simulink model "gm_uz_pmsm_model_9ph_working_vnl"  (R2021a)
settings: Solver=FixedStepAuto  StartTime=0.0  StopTime=0.04  RelTol=1e-3
PreLoadFcn:
  | uz_pmsm_model_9ph_init_parameter
undefined symbols (not defined in the file or in its folder): a, b, c, friction_coefficient, inertia, k_i_d, k_p_d, k_p_q, L_d, L_o1, L_o2, L_q, L_x1, L_x2, L_y1, L_y2, L_zero, polepair, psi_pm, R_1, static_friction_torque, ts
libraries: hdlmdlgenlib x182, hdlsllib x92, simulink x15, pid_lib x2
(part 4 of 5)

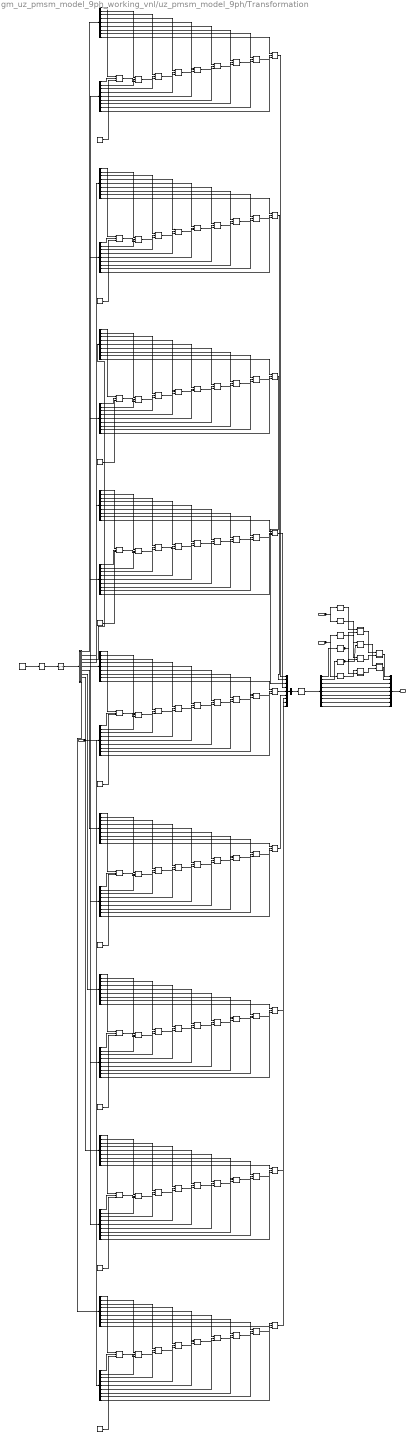
== system gm_uz_pmsm_model_9ph_working_vnl/uz_pmsm_model_9ph/Transformation ==
  in : Inport  OutDataTypeStr=fixdt(1, 25, 12)  PortDimensions=[9]  SampleTime=2e-09
  sin_theta_el : Inport  Port=2  OutDataTypeStr=single  SampleTime=2e-09
  cos_theta_el : Inport  Port=3  OutDataTypeStr=single  SampleTime=2e-09
  Add : Subsystem
      mask Display: disp('NFP\nadd');
  Add1 : Subsystem
      mask Display: disp('NFP\nadd');
  Constant1 : Constant  Value=[0.22222137451171875;0;0.22222137451171875;0;0.22222137451171875;0;0.22222137451171875;0;0.111110687255859375;-0.111110687255859375;0.1924495697021484375;0.22222137451171875;0;-0.111110687255859375;-0.1924495697021484375;-0.111110687255859375;0.1924495697021484375;0.111110687255859375;-0.111110687255859375;-0.1924495697021484375;0.22222137451171875;0;-0.111110687255859375;0.1924495697021484375;-0.111110687255859375;-0.1924495697021484375;0.111110687255859375;0.208820343017578125;0.0760040283203125;0.111110687255859375;0.1924495697021484375;-0.0385875701904296875;0.218845367431640625;-0.1702327728271484375;0.142841339111328125;-0.111110687255859375;-0.1702327728271484375;0.142841339111328125;0.111110687255859375;0.1924495697021484375;0.208820343017578125;-0.0760040283203125;-0.0385875701904296875;-0.218845367431640625;-0.111110687255859375;-0.0385875701904296875;-0.218845367431640625;0.111110687255859375;0.1924495697021484375;-0.1702327728271484375;-0.142841339111328125;0.208820343017578125;0.0760040283203125;-0.111110687255859375;0.1702327728271484375;0.142841339111328125;-0.111110687255859375;0.1924495697021484375;-0.208820343017578125;-0.0760040283203125;0.0385875701904296875;-0.218845367431640625;0.111110687255859375;-0.208820343017578125;0.0760040283203125;-0.111110687255859375;0.1924495697021484375;0.0385875701904296875;0.218845367431640625;0.1702327728271484375;0.142841339111328125;0.111110687255859375;0.0385875701904296875;-0.218845367431640625;-0.111110687255859375;0.1924495697021484375;0.1702327728271484375;-0.142841339111328125;-0.208820343017578125;0.0760040283203125;0.111110687255859375]  OutDataTypeStr=fixdt(1, 18, 19)  SampleTime=2e-09
  Data Type Conversion39 : Subsystem
      mask Display: disp('NFP\nconv');
  Data Type Conversion39_out1_0_wire : hdlmdlgenlib/Buffer
      settings: SourceProductBaseCode=SL
  Data Type Conversion39_out1_1_wire : hdlmdlgenlib/Buffer
      settings: SourceProductBaseCode=SL
  Divide : Subsystem
      mask Display: disp('NFP\nmul');
  Divide1 : Subsystem
      mask Display: disp('NFP\nmul');
  Divide2 : Subsystem
      mask Display: disp('NFP\nmul');
  Divide3 : Subsystem
      mask Display: disp('NFP\nmul');
  From{1..2,17..18} (4 alike) : hdlmdlgenlib/Buffer
      settings: SourceProductBaseCode=SL
  _adder_MultiplyAdd{,1..80} (81 alike) : hdlsllib/HDL Operations/Multiply-Add  Function=c+(a.*b)  datatype=fixdt(1, 43, 31)  DoSatur=off  FMA=off
      settings: SourceProductBaseCode=SL
  _bias{,1..8} (9 alike) : Constant  Value=double(0)  OutDataTypeStr=fixdt(1, 43, 31)  SampleTime=2e-09
  mux : Mux  Inputs=9
  t{,6..23} (19 alike) : Demux  Outputs=9
  t1 : Reshape  OutputDimensionality=Customize  OutputDimensions=[9,9]
  t2 : Math  Operator=transpose  SaturateOnIntegerOverflow=on
  t3 : Subsystem
  t4 : Mux  Inputs=9
  t5 : Concatenate  NumInputs=1  Mode=Multidimensional array  ConcatenateDimension=2
  out : Outport  SampleTime=2e-09
  wires:
  cos_theta_el/1 -> From17/1, From2/1
  sin_theta_el/1 -> From1/1, From18/1
  in/1 -> t7/1, t9/1, t11/1, t13/1, t15/1, t17/1, t19/1, t21/1, t23/1
  From1/1 -> Divide2/1(In1)
  From2/1 -> Divide3/1(In1)
  From18/1 -> Divide1/1(In1)
  From17/1 -> Divide/1(In1)
  Divide3/1(Out1) -> Add1/1(In1)
  Divide2/1(Out1) -> Add1/2(In2)
  Divide1/1(Out1) -> Add/2(In2)
  Divide/1(Out1) -> Add/1(In1)
  Data Type Conversion39/1(Out1) -> t/1
  Add1/1(Out1) -> mux/2
  Add/1(Out1) -> mux/1
  _adder_MultiplyAdd79/1 -> _adder_MultiplyAdd80/3
  t23/9 -> _adder_MultiplyAdd80/2
  t22/9 -> _adder_MultiplyAdd80/1
  _adder_MultiplyAdd78/1 -> _adder_MultiplyAdd79/3
  t23/8 -> _adder_MultiplyAdd79/2
  t22/8 -> _adder_MultiplyAdd79/1
  _adder_MultiplyAdd77/1 -> _adder_MultiplyAdd78/3
  t23/7 -> _adder_MultiplyAdd78/2
  t22/7 -> _adder_MultiplyAdd78/1
  _adder_MultiplyAdd76/1 -> _adder_MultiplyAdd77/3
  t23/6 -> _adder_MultiplyAdd77/2
  t22/6 -> _adder_MultiplyAdd77/1
  _adder_MultiplyAdd75/1 -> _adder_MultiplyAdd76/3
  t23/5 -> _adder_MultiplyAdd76/2
  t22/5 -> _adder_MultiplyAdd76/1
  _adder_MultiplyAdd74/1 -> _adder_MultiplyAdd75/3
  t23/4 -> _adder_MultiplyAdd75/2
  t22/4 -> _adder_MultiplyAdd75/1
  _adder_MultiplyAdd73/1 -> _adder_MultiplyAdd74/3
  t23/3 -> _adder_MultiplyAdd74/2
  t22/3 -> _adder_MultiplyAdd74/1
  _adder_MultiplyAdd72/1 -> _adder_MultiplyAdd73/3
  t23/2 -> _adder_MultiplyAdd73/2
  t22/2 -> _adder_MultiplyAdd73/1
  t23/1 -> _adder_MultiplyAdd72/2
  t22/1 -> _adder_MultiplyAdd72/1
  _bias8/1 -> _adder_MultiplyAdd72/3
  _adder_MultiplyAdd70/1 -> _adder_MultiplyAdd71/3
  t21/9 -> _adder_MultiplyAdd71/2
  t20/9 -> _adder_MultiplyAdd71/1
  _adder_MultiplyAdd69/1 -> _adder_MultiplyAdd70/3
  t21/8 -> _adder_MultiplyAdd70/2
  t20/8 -> _adder_MultiplyAdd70/1
  _adder_MultiplyAdd68/1 -> _adder_MultiplyAdd69/3
  t21/7 -> _adder_MultiplyAdd69/2
  t20/7 -> _adder_MultiplyAdd69/1
  _adder_MultiplyAdd67/1 -> _adder_MultiplyAdd68/3
  t21/6 -> _adder_MultiplyAdd68/2
  t20/6 -> _adder_MultiplyAdd68/1
  _adder_MultiplyAdd66/1 -> _adder_MultiplyAdd67/3
  t21/5 -> _adder_MultiplyAdd67/2
  t20/5 -> _adder_MultiplyAdd67/1
  _adder_MultiplyAdd65/1 -> _adder_MultiplyAdd66/3
  t21/4 -> _adder_MultiplyAdd66/2
  t20/4 -> _adder_MultiplyAdd66/1
  _adder_MultiplyAdd64/1 -> _adder_MultiplyAdd65/3
  t21/3 -> _adder_MultiplyAdd65/2
  t20/3 -> _adder_MultiplyAdd65/1
  _adder_MultiplyAdd63/1 -> _adder_MultiplyAdd64/3
  t21/2 -> _adder_MultiplyAdd64/2
  t20/2 -> _adder_MultiplyAdd64/1
  t21/1 -> _adder_MultiplyAdd63/2
  t20/1 -> _adder_MultiplyAdd63/1
  _bias7/1 -> _adder_MultiplyAdd63/3
  _adder_MultiplyAdd61/1 -> _adder_MultiplyAdd62/3
  t19/9 -> _adder_MultiplyAdd62/2
  t18/9 -> _adder_MultiplyAdd62/1
  _adder_MultiplyAdd60/1 -> _adder_MultiplyAdd61/3
  t19/8 -> _adder_MultiplyAdd61/2
  t18/8 -> _adder_MultiplyAdd61/1
  _adder_MultiplyAdd59/1 -> _adder_MultiplyAdd60/3
  t19/7 -> _adder_MultiplyAdd60/2
  t18/7 -> _adder_MultiplyAdd60/1
  _adder_MultiplyAdd58/1 -> _adder_MultiplyAdd59/3
  t19/6 -> _adder_MultiplyAdd59/2
  t18/6 -> _adder_MultiplyAdd59/1
  _adder_MultiplyAdd57/1 -> _adder_MultiplyAdd58/3
  t19/5 -> _adder_MultiplyAdd58/2
  t18/5 -> _adder_MultiplyAdd58/1
  _adder_MultiplyAdd56/1 -> _adder_MultiplyAdd57/3
  t19/4 -> _adder_MultiplyAdd57/2
  t18/4 -> _adder_MultiplyAdd57/1
  _adder_MultiplyAdd55/1 -> _adder_MultiplyAdd56/3
  t19/3 -> _adder_MultiplyAdd56/2
  t18/3 -> _adder_MultiplyAdd56/1
  _adder_MultiplyAdd54/1 -> _adder_MultiplyAdd55/3
  t19/2 -> _adder_MultiplyAdd55/2
  t18/2 -> _adder_MultiplyAdd55/1
  t19/1 -> _adder_MultiplyAdd54/2
  t18/1 -> _adder_MultiplyAdd54/1
  _bias6/1 -> _adder_MultiplyAdd54/3
  _adder_MultiplyAdd52/1 -> _adder_MultiplyAdd53/3
  t17/9 -> _adder_MultiplyAdd53/2
  t16/9 -> _adder_MultiplyAdd53/1
  _adder_MultiplyAdd51/1 -> _adder_MultiplyAdd52/3
  t17/8 -> _adder_MultiplyAdd52/2
  t16/8 -> _adder_MultiplyAdd52/1
  _adder_MultiplyAdd50/1 -> _adder_MultiplyAdd51/3
  t17/7 -> _adder_MultiplyAdd51/2
  t16/7 -> _adder_MultiplyAdd51/1
  _adder_MultiplyAdd49/1 -> _adder_MultiplyAdd50/3
  t17/6 -> _adder_MultiplyAdd50/2
  t16/6 -> _adder_MultiplyAdd50/1
  _adder_MultiplyAdd48/1 -> _adder_MultiplyAdd49/3
  t17/5 -> _adder_MultiplyAdd49/2
  t16/5 -> _adder_MultiplyAdd49/1
  _adder_MultiplyAdd47/1 -> _adder_MultiplyAdd48/3
  t17/4 -> _adder_MultiplyAdd48/2
  t16/4 -> _adder_MultiplyAdd48/1
  _adder_MultiplyAdd46/1 -> _adder_MultiplyAdd47/3
  t17/3 -> _adder_MultiplyAdd47/2
  t16/3 -> _adder_MultiplyAdd47/1
  _adder_MultiplyAdd45/1 -> _adder_MultiplyAdd46/3
  t17/2 -> _adder_MultiplyAdd46/2
  t16/2 -> _adder_MultiplyAdd46/1
  t17/1 -> _adder_MultiplyAdd45/2
  t16/1 -> _adder_MultiplyAdd45/1
  _bias5/1 -> _adder_MultiplyAdd45/3
  _adder_MultiplyAdd43/1 -> _adder_MultiplyAdd44/3
  t15/9 -> _adder_MultiplyAdd44/2
  t14/9 -> _adder_MultiplyAdd44/1
  _adder_MultiplyAdd42/1 -> _adder_MultiplyAdd43/3
  t15/8 -> _adder_MultiplyAdd43/2
  t14/8 -> _adder_MultiplyAdd43/1
  _adder_MultiplyAdd41/1 -> _adder_MultiplyAdd42/3
  t15/7 -> _adder_MultiplyAdd42/2
  t14/7 -> _adder_MultiplyAdd42/1
  _adder_MultiplyAdd40/1 -> _adder_MultiplyAdd41/3
  t15/6 -> _adder_MultiplyAdd41/2
  t14/6 -> _adder_MultiplyAdd41/1
  _adder_MultiplyAdd39/1 -> _adder_MultiplyAdd40/3
  t15/5 -> _adder_MultiplyAdd40/2
  t14/5 -> _adder_MultiplyAdd40/1
  _adder_MultiplyAdd38/1 -> _adder_MultiplyAdd39/3
  t15/4 -> _adder_MultiplyAdd39/2
  t14/4 -> _adder_MultiplyAdd39/1
  _adder_MultiplyAdd37/1 -> _adder_MultiplyAdd38/3
  t15/3 -> _adder_MultiplyAdd38/2
  t14/3 -> _adder_MultiplyAdd38/1
  _adder_MultiplyAdd36/1 -> _adder_MultiplyAdd37/3
  t15/2 -> _adder_MultiplyAdd37/2
  t14/2 -> _adder_MultiplyAdd37/1
  t15/1 -> _adder_MultiplyAdd36/2
  t14/1 -> _adder_MultiplyAdd36/1
  _bias4/1 -> _adder_MultiplyAdd36/3
  _adder_MultiplyAdd34/1 -> _adder_MultiplyAdd35/3
  t13/9 -> _adder_MultiplyAdd35/2
  t12/9 -> _adder_MultiplyAdd35/1
  _adder_MultiplyAdd33/1 -> _adder_MultiplyAdd34/3
  t13/8 -> _adder_MultiplyAdd34/2
  t12/8 -> _adder_MultiplyAdd34/1
  _adder_MultiplyAdd32/1 -> _adder_MultiplyAdd33/3
  t13/7 -> _adder_MultiplyAdd33/2
  t12/7 -> _adder_MultiplyAdd33/1
  _adder_MultiplyAdd31/1 -> _adder_MultiplyAdd32/3
  t13/6 -> _adder_MultiplyAdd32/2
  t12/6 -> _adder_MultiplyAdd32/1
  _adder_MultiplyAdd30/1 -> _adder_MultiplyAdd31/3
  t13/5 -> _adder_MultiplyAdd31/2
  t12/5 -> _adder_MultiplyAdd31/1
  _adder_MultiplyAdd29/1 -> _adder_MultiplyAdd30/3
  t13/4 -> _adder_MultiplyAdd30/2
  t12/4 -> _adder_MultiplyAdd30/1
  _adder_MultiplyAdd28/1 -> _adder_MultiplyAdd29/3
  t13/3 -> _adder_MultiplyAdd29/2
  t12/3 -> _adder_MultiplyAdd29/1
  _adder_MultiplyAdd27/1 -> _adder_MultiplyAdd28/3
  t13/2 -> _adder_MultiplyAdd28/2
  t12/2 -> _adder_MultiplyAdd28/1
  t13/1 -> _adder_MultiplyAdd27/2
  t12/1 -> _adder_MultiplyAdd27/1
  _bias3/1 -> _adder_MultiplyAdd27/3
  _adder_MultiplyAdd25/1 -> _adder_MultiplyAdd26/3
  t11/9 -> _adder_MultiplyAdd26/2
  t10/9 -> _adder_MultiplyAdd26/1
  _adder_MultiplyAdd24/1 -> _adder_MultiplyAdd25/3
  t11/8 -> _adder_MultiplyAdd25/2
  t10/8 -> _adder_MultiplyAdd25/1
  _adder_MultiplyAdd23/1 -> _adder_MultiplyAdd24/3
  t11/7 -> _adder_MultiplyAdd24/2
  t10/7 -> _adder_MultiplyAdd24/1
  _adder_MultiplyAdd22/1 -> _adder_MultiplyAdd23/3
  t11/6 -> _adder_MultiplyAdd23/2
  t10/6 -> _adder_MultiplyAdd23/1
  _adder_MultiplyAdd21/1 -> _adder_MultiplyAdd22/3
  t11/5 -> _adder_MultiplyAdd22/2
  t10/5 -> _adder_MultiplyAdd22/1
  _adder_MultiplyAdd20/1 -> _adder_MultiplyAdd21/3
  t11/4 -> _adder_MultiplyAdd21/2
  t10/4 -> _adder_MultiplyAdd21/1
  _adder_MultiplyAdd19/1 -> _adder_MultiplyAdd20/3
  t11/3 -> _adder_MultiplyAdd20/2
  t10/3 -> _adder_MultiplyAdd20/1
  _adder_MultiplyAdd18/1 -> _adder_MultiplyAdd19/3
  t11/2 -> _adder_MultiplyAdd19/2
  t10/2 -> _adder_MultiplyAdd19/1
  t11/1 -> _adder_MultiplyAdd18/2
  t10/1 -> _adder_MultiplyAdd18/1
  _bias2/1 -> _adder_MultiplyAdd18/3
  _adder_MultiplyAdd16/1 -> _adder_MultiplyAdd17/3
  t9/9 -> _adder_MultiplyAdd17/2
  t8/9 -> _adder_MultiplyAdd17/1
  _adder_MultiplyAdd15/1 -> _adder_MultiplyAdd16/3
  t9/8 -> _adder_MultiplyAdd16/2
  t8/8 -> _adder_MultiplyAdd16/1
  _adder_MultiplyAdd14/1 -> _adder_MultiplyAdd15/3
  t9/7 -> _adder_MultiplyAdd15/2
  t8/7 -> _adder_MultiplyAdd15/1
  _adder_MultiplyAdd13/1 -> _adder_MultiplyAdd14/3
  t9/6 -> _adder_MultiplyAdd14/2
  t8/6 -> _adder_MultiplyAdd14/1
  _adder_MultiplyAdd12/1 -> _adder_MultiplyAdd13/3
  t9/5 -> _adder_MultiplyAdd13/2
  t8/5 -> _adder_MultiplyAdd13/1
  _adder_MultiplyAdd11/1 -> _adder_MultiplyAdd12/3
  t9/4 -> _adder_MultiplyAdd12/2
  t8/4 -> _adder_MultiplyAdd12/1
  _adder_MultiplyAdd10/1 -> _adder_MultiplyAdd11/3
  t9/3 -> _adder_MultiplyAdd11/2
  t8/3 -> _adder_MultiplyAdd11/1
  _adder_MultiplyAdd9/1 -> _adder_MultiplyAdd10/3
  t9/2 -> _adder_MultiplyAdd10/2
  t8/2 -> _adder_MultiplyAdd10/1
  t9/1 -> _adder_MultiplyAdd9/2
  t8/1 -> _adder_MultiplyAdd9/1
  _bias1/1 -> _adder_MultiplyAdd9/3
  _adder_MultiplyAdd7/1 -> _adder_MultiplyAdd8/3
  t7/9 -> _adder_MultiplyAdd8/2
  t6/9 -> _adder_MultiplyAdd8/1
  _adder_MultiplyAdd6/1 -> _adder_MultiplyAdd7/3
  t7/8 -> _adder_MultiplyAdd7/2
  t6/8 -> _adder_MultiplyAdd7/1
  _adder_MultiplyAdd5/1 -> _adder_MultiplyAdd6/3
  t7/7 -> _adder_MultiplyAdd6/2
  t6/7 -> _adder_MultiplyAdd6/1
  _adder_MultiplyAdd4/1 -> _adder_MultiplyAdd5/3
  t7/6 -> _adder_MultiplyAdd5/2
  t6/6 -> _adder_MultiplyAdd5/1
  _adder_MultiplyAdd3/1 -> _adder_MultiplyAdd4/3
  t7/5 -> _adder_MultiplyAdd4/2
  t6/5 -> _adder_MultiplyAdd4/1
  _adder_MultiplyAdd2/1 -> _adder_MultiplyAdd3/3
  t7/4 -> _adder_MultiplyAdd3/2
  t6/4 -> _adder_MultiplyAdd3/1
  _adder_MultiplyAdd1/1 -> _adder_MultiplyAdd2/3
  t7/3 -> _adder_MultiplyAdd2/2
  t6/3 -> _adder_MultiplyAdd2/1
  _adder_MultiplyAdd/1 -> _adder_MultiplyAdd1/3
  t7/2 -> _adder_MultiplyAdd1/2
  t6/2 -> _adder_MultiplyAdd1/1
  t7/1 -> _adder_MultiplyAdd/2
  t6/1 -> _adder_MultiplyAdd/1
  _bias/1 -> _adder_MultiplyAdd/3
  t4/1 -> t5/1
  _adder_MultiplyAdd80/1 -> t4/9
  _adder_MultiplyAdd71/1 -> t4/8
  _adder_MultiplyAdd62/1 -> t4/7
  _adder_MultiplyAdd53/1 -> t4/6
  _adder_MultiplyAdd44/1 -> t4/5
  _adder_MultiplyAdd35/1 -> t4/4
  _adder_MultiplyAdd26/1 -> t4/3
  _adder_MultiplyAdd17/1 -> t4/2
  _adder_MultiplyAdd8/1 -> t4/1
  t3/9(out8) -> t22/1
  t3/8(out7) -> t20/1
  t3/7(out6) -> t18/1
  t3/6(out5) -> t16/1
  t3/5(out4) -> t14/1
  t3/4(out3) -> t12/1
  t3/3(out2) -> t10/1
  t3/2(out1) -> t8/1
  t3/1(out0) -> t6/1
  t2/1 -> t3/1(in0)
  Constant1/1 -> t1/1
  t/9 -> mux/9
  t/8 -> mux/8
  t/7 -> mux/7
  t/6 -> mux/6
  t/5 -> mux/5
  t/4 -> mux/4
  t/3 -> mux/3
  t/2 -> Data Type Conversion39_out1_1_wire/1
  t/1 -> Data Type Conversion39_out1_0_wire/1
  mux/1 -> out/1
  t5/1 -> Data Type Conversion39/1(In1)
  Data Type Conversion39_out1_1_wire/1 -> Divide1/2(In2), Divide3/2(In2)
  Data Type Conversion39_out1_0_wire/1 -> Divide/2(In2), Divide2/2(In2)
  t1/1 -> t2/1

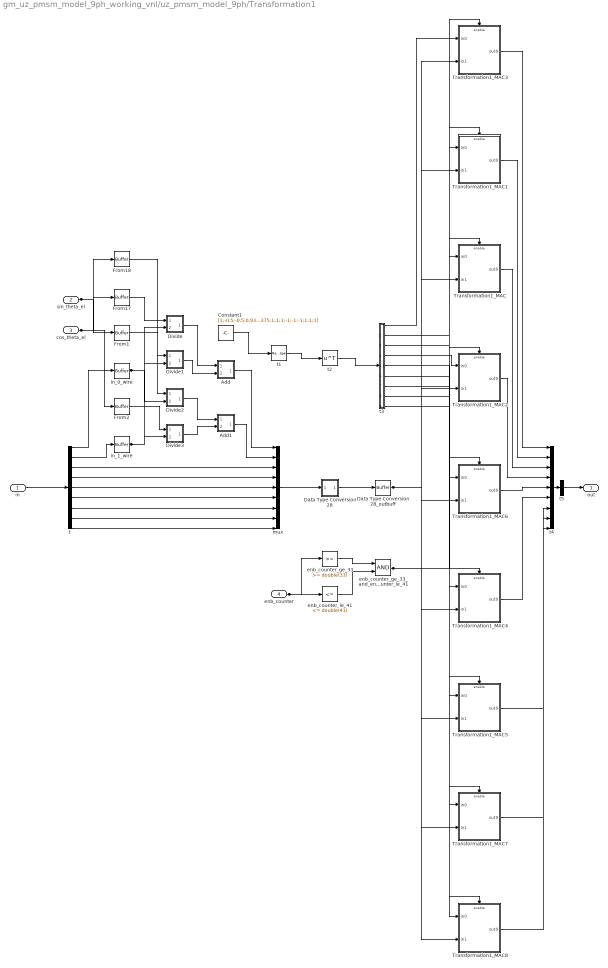
== system gm_uz_pmsm_model_9ph_working_vnl/uz_pmsm_model_9ph/Transformation1 ==
  in : Inport  OutDataTypeStr=single  PortDimensions=[9]  SampleTime=2e-09
  sin_theta_el : Inport  Port=2  OutDataTypeStr=single  SampleTime=2e-09
  cos_theta_el : Inport  Port=3  OutDataTypeStr=single  SampleTime=2e-09
  enb_counter : Inport  Port=4  OutDataTypeStr=uint16  SampleTime=2e-09
  Add : Subsystem
      mask Display: disp('NFP\nadd');
  Add1 : Subsystem
      mask Display: disp('NFP\nadd');
  Constant1 : Constant  Value=[1;-0.5;-0.5;0.939697265625;-0.7660369873046875;-0.17364501953125;0.7660369873046875;-0.939697265625;0.17364501953125;0;0.86602783203125;-0.86602783203125;0.3420257568359375;0.642791748046875;-0.98480224609375;0.642791748046875;0.3420257568359375;-0.98480224609375;1;1;1;0.5;0.5;0.5;-0.5;-0.5;-0.5;0;0;0;0.86602783203125;0.86602783203125;0.86602783203125;0.86602783203125;0.86602783203125;0.86602783203125;1;-0.5;-0.5;-0.17364501953125;0.939697265625;-0.7660369873046875;-0.939697265625;0.17364501953125;0.7660369873046875;0;-0.86602783203125;0.86602783203125;0.98480224609375;-0.3420257568359375;-0.642791748046875;-0.3420257568359375;0.98480224609375;-0.642791748046875;1;-0.5;-0.5;-0.7660369873046875;-0.17364501953125;0.939697265625;0.17364501953125;0.7660369873046875;-0.939697265625;0;0.86602783203125;-0.86602783203125;0.642791748046875;-0.98480224609375;0.3420257568359375;-0.98480224609375;0.642791748046875;0.3420257568359375;1;1;1;-1;-1;-1;1;1;1]  OutDataTypeStr=fixdt(1, 18, 16)  SampleTime=2e-09
  Data Type Conversion28 : Subsystem
      mask Display: disp('NFP\nconv');
  Data Type Conversion28_outbuff : hdlmdlgenlib/Buffer
      settings: SourceProductBaseCode=SL
  Divide : Subsystem
      mask Display: disp('NFP\nmul');
  Divide1 : Subsystem
      mask Display: disp('NFP\nmul');
  Divide2 : Subsystem
      mask Display: disp('NFP\nmul');
  Divide3 : Subsystem
      mask Display: disp('NFP\nmul');
  From{1..2,17..18} (4 alike) : hdlmdlgenlib/Buffer
      settings: SourceProductBaseCode=SL
  Transformation1_MAC : Subsystem
      settings: MinAlgLoopOccurrences=on
  Transformation1_MAC1 : Subsystem
      settings: MinAlgLoopOccurrences=on
  Transformation1_MAC2 : Subsystem
      settings: MinAlgLoopOccurrences=on
  Transformation1_MAC3 : Subsystem
      settings: MinAlgLoopOccurrences=on
  Transformation1_MAC4 : Subsystem
      settings: MinAlgLoopOccurrences=on
  Transformation1_MAC5 : Subsystem
      settings: MinAlgLoopOccurrences=on
  Transformation1_MAC6 : Subsystem
      settings: MinAlgLoopOccurrences=on
  Transformation1_MAC7 : Subsystem
      settings: MinAlgLoopOccurrences=on
  Transformation1_MAC8 : Subsystem
      settings: MinAlgLoopOccurrences=on
  enb_counter_ge_33 : simulink/Logic and Bit Operations/Compare To Constant  relop=>=  const=double(33)  OutDataTypeStr=boolean
  enb_counter_ge_33_and_enb_counter_le_41 : Logic  AllPortsSameDT=off  OutDataTypeStr=boolean  SampleTime=2e-09
  enb_counter_le_41 : simulink/Logic and Bit Operations/Compare To Constant  relop=<=  const=double(41)  OutDataTypeStr=boolean
  in_0_wire : hdlmdlgenlib/Buffer
      settings: SourceProductBaseCode=SL
  in_1_wire : hdlmdlgenlib/Buffer
      settings: SourceProductBaseCode=SL
  mux : Mux  Inputs=9
  t : Demux  Outputs=9
  t1 : Reshape  OutputDimensionality=Customize  OutputDimensions=[9,9]
  t2 : Math  Operator=transpose  SaturateOnIntegerOverflow=on
  t3 : Subsystem
  t4 : Mux  Inputs=9
  t5 : Concatenate  NumInputs=1  Mode=Multidimensional array  ConcatenateDimension=2
  out : Outport  SampleTime=2e-09
  wires:
  enb_counter/1 -> enb_counter_ge_33/1, enb_counter_le_41/1
  cos_theta_el/1 -> From17/1, From2/1
  sin_theta_el/1 -> From1/1, From18/1
  in/1 -> t/1
  enb_counter_le_41/1 -> enb_counter_ge_33_and_enb_counter_le_41/2
  enb_counter_ge_33/1 -> enb_counter_ge_33_and_enb_counter_le_41/1
  enb_counter_ge_33_and_enb_counter_le_41/1 -> Transformation1_MAC8/Enable, Transformation1_MAC7/Enable, Transformation1_MAC5/Enable, Transformation1_MAC4/Enable, Transformation1_MAC6/Enable, Transformation1_MAC2/Enable, Transformation1_MAC/Enable, Transformation1_MAC1/Enable, Transformation1_MAC3/Enable
  t3/9(out8) -> Transformation1_MAC8/1(in0)
  t3/8(out7) -> Transformation1_MAC7/1(in0)
  t3/7(out6) -> Transformation1_MAC5/1(in0)
  t3/6(out5) -> Transformation1_MAC4/1(in0)
  t3/5(out4) -> Transformation1_MAC6/1(in0)
  t3/4(out3) -> Transformation1_MAC2/1(in0)
  t3/3(out2) -> Transformation1_MAC/1(in0)
  t3/2(out1) -> Transformation1_MAC1/1(in0)
  t3/1(out0) -> Transformation1_MAC3/1(in0)
  Divide3/1(Out1) -> Add1/2(In2)
  Divide2/1(Out1) -> Add1/1(In1)
  Divide1/1(Out1) -> Add/2(In2)
  Divide/1(Out1) -> Add/1(In1)
  Data Type Conversion28/1(Out1) -> Data Type Conversion28_outbuff/1
  Add1/1(Out1) -> mux/2
  Add/1(Out1) -> mux/1
  t4/1 -> t5/1
  Transformation1_MAC8/1(out0) -> t4/9
  Transformation1_MAC7/1(out0) -> t4/8
  Transformation1_MAC5/1(out0) -> t4/7
  Transformation1_MAC4/1(out0) -> t4/6
  Transformation1_MAC6/1(out0) -> t4/5
  Transformation1_MAC2/1(out0) -> t4/4
  Transformation1_MAC/1(out0) -> t4/3
  Transformation1_MAC1/1(out0) -> t4/2
  Transformation1_MAC3/1(out0) -> t4/1
  t2/1 -> t3/1(in0)
  Constant1/1 -> t1/1
  t/9 -> mux/9
  t/8 -> mux/8
  t/7 -> mux/7
  t/6 -> mux/6
  t/5 -> mux/5
  t/4 -> mux/4
  t/3 -> mux/3
  t/2 -> in_1_wire/1
  t/1 -> in_0_wire/1
  mux/1 -> Data Type Conversion28/1(In1)
  t5/1 -> out/1
  From2/1 -> Divide3/1(In1)
  From18/1 -> Divide1/1(In1)
  From17/1 -> Divide/1(In1)
  From1/1 -> Divide2/1(In1)
  in_1_wire/1 -> Divide1/2(In2), Divide3/2(In2)
  in_0_wire/1 -> Divide/2(In2), Divide2/2(In2)
  Data Type Conversion28_outbuff/1 -> Transformation1_MAC8/2(in1), Transformation1_MAC7/2(in1), Transformation1_MAC5/2(in1), Transformation1_MAC4/2(in1), Transformation1_MAC6/2(in1), Transformation1_MAC2/2(in1), Transformation1_MAC/2(in1), Transformation1_MAC1/2(in1), Transformation1_MAC3/2(in1)
  t1/1 -> t2/1

== system gm_uz_pmsm_model_9ph_working_vnl/uz_pmsm_model_9ph_vnl/Theta_el ==
  w_mech : Inport
  polepairs : Inport  Port=2
  reset : Inport  Port=3
  Data Type Conversion1 : DataTypeConversion  OutDataTypeStr=single  RndMeth=Nearest
  Data Type Conversion2 : DataTypeConversion  OutDataTypeStr=double  RndMeth=Nearest
  Divide : Product  Inputs=**
  Mod : Math  Operator=rem  SaturateOnIntegerOverflow=on
  Pi : Constant  Value=2*pi  OutDataTypeStr=single  SampleTime=-1
  integrator8 : Subsystem
  theta_el : Outport
  wires:
  Data Type Conversion2/1 -> integrator8/1(in)
  Mod/1 -> theta_el/1  "theta_el"
  Data Type Conversion1/1 -> Mod/1
  Pi/1 -> Mod/2
  reset/1 -> integrator8/2(reset)
  integrator8/1(outt) -> Data Type Conversion1/1
  polepairs/1 -> Divide/2
  w_mech/1 -> Divide/1
  Divide/1 -> Data Type Conversion2/1

== system gm_uz_pmsm_model_9ph_working_vnl/uz_pmsm_model_9ph_vnl/Transformation ==
  in : Inport
  Add : Sum
  Add1 : Sum  Inputs=-+
  Constant1 : Constant  Value=c  OutDataTypeStr=fixdt(1,18)  SampleTime=-1
  Data Type Conversion1 : DataTypeConversion  OutDataTypeStr=single  RndMeth=Nearest
  Data Type Conversion38 : DataTypeConversion  OutDataTypeStr=single  RndMeth=Nearest
  Data Type Conversion39 : DataTypeConversion  OutDataTypeStr=single  RndMeth=Nearest
  Demux1 : Demux  Outputs=9
  Divide{,1..3} (4 alike) : Product  Inputs=**
  MatrixMultiply : Product  Multiplication=Matrix(*)
  Mux : Mux  Inputs=9
  out : Outport
  wires:
  in/1 -> MatrixMultiply/2
  Data Type Conversion39/1 -> Demux1/1
  Constant1/1 -> MatrixMultiply/1
  MatrixMultiply/1 -> Data Type Conversion39/1
  Divide2/1 -> Add1/1
  Divide3/1 -> Add1/2
  [cos_theta_el] -> Divide3/1
  [sin_theta_el] -> Divide2/1
  [cos_theta_el] -> Divide/1
  [sin_theta_el] -> Divide1/1
  Divide1/1 -> Add/2
  Divide/1 -> Add/1
  Data Type Conversion1/1 -> Divide3/2, Divide1/2  "u_beta"
  Data Type Conversion38/1 -> Divide2/2, Divide/2  "u_alpha"
  Add/1 -> Mux/1
  Add1/1 -> Mux/2
  Demux1/2 -> Data Type Conversion1/1
  Demux1/1 -> Data Type Conversion38/1
  Mux/1 -> out/1
  Demux1/9 -> Mux/9
  Demux1/8 -> Mux/8
  Demux1/7 -> Mux/7
  Demux1/6 -> Mux/6
  Demux1/5 -> Mux/5
  Demux1/4 -> Mux/4
  Demux1/3 -> Mux/3

== system gm_uz_pmsm_model_9ph_working_vnl/uz_pmsm_model_9ph_vnl/Transformation1 ==
  in : Inport
  Add : Sum  Inputs=+-
  Add1 : Sum
  Constant1 : Constant  Value=inv(c)  OutDataTypeStr=fixdt(1,18)  SampleTime=-1
  Data Type Conversion28 : DataTypeConversion  OutDataTypeStr=fixdt(1,25,12)  RndMeth=Nearest
  Demux1 : Demux  Outputs=9
  Divide{,1..3} (4 alike) : Product  Inputs=**
  MatrixMultiply : Product  Multiplication=Matrix(*)
  Mux : Mux  Inputs=9
  out : Outport
  wires:
  MatrixMultiply/1 -> out/1
  Constant1/1 -> MatrixMultiply/1
  Data Type Conversion28/1 -> MatrixMultiply/2
  Add1/1 -> Mux/2
  [cos_theta_el] -> Divide3/1
  Divide2/1 -> Add1/1
  [sin_theta_el] -> Divide2/1
  Divide3/1 -> Add1/2
  Demux1/1 -> Divide/2, Divide2/2  "i_d"
  Divide1/1 -> Add/2
  [cos_theta_el] -> Divide/1
  Divide/1 -> Add/1
  Add/1 -> Mux/1
  Demux1/2 -> Divide1/2, Divide3/2  "i_q"
  [sin_theta_el] -> Divide1/1
  Demux1/7 -> Mux/7
  Demux1/9 -> Mux/9
  Demux1/5 -> Mux/5
  Demux1/3 -> Mux/3
  Demux1/4 -> Mux/4
  Demux1/6 -> Mux/6
  Demux1/8 -> Mux/8
  Mux/1 -> Data Type Conversion28/1
  in/1 -> Demux1/1

== system gm_uz_pmsm_model_9ph_working_vnl/uz_pmsm_model_9ph_vnl/mechanical_system ==
  note: This delay breaks the algebraic loop between mechanical and electrical system.
      | Introduces a delay of 500ns.
  reset : Inport
  M_Mi : Inport  Port=2
  reciprocal_J : Inport  Port=3
  load_torque : Inport  Port=4
  Data Type Conversion1 : DataTypeConversion  OutDataTypeStr=double  RndMeth=Nearest
  Data Type Conversion8 : DataTypeConversion  OutDataTypeStr=single  RndMeth=Nearest
  Delay : Delay  DelayLength=1
  Product11 : Product
  Sum1 : Sum  Inputs=|+-
  integrator1 : Subsystem
  omega_mech : Outport
  wires:
  Data Type Conversion1/1 -> integrator1/2(in)
  Data Type Conversion8/1 -> omega_mech/1
  Delay/1 -> Sum1/1
  M_Mi/1 -> Delay/1
  load_torque/1 -> Sum1/2
  Sum1/1 -> Product11/2
  reciprocal_J/1 -> Product11/1
  reset/1 -> integrator1/1(reset)
  integrator1/1(outt) -> Data Type Conversion8/1
  Product11/1 -> Data Type Conversion1/1

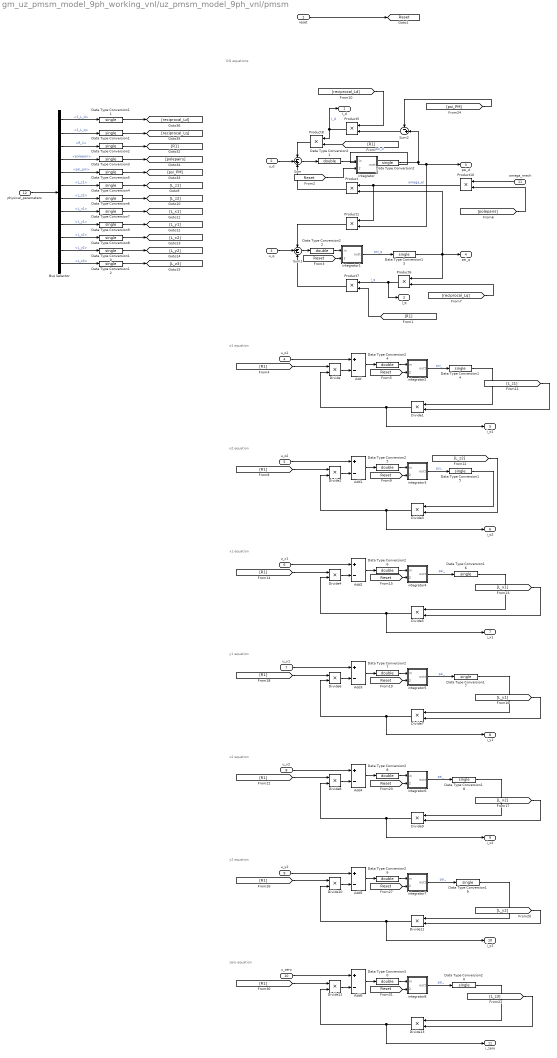
== system gm_uz_pmsm_model_9ph_working_vnl/uz_pmsm_model_9ph_vnl/pmsm ==
  note: zero equation
  note: y2 equation
  note: x2 equation
  note: y1 equation
  note: x1 equation
  note: o2 equation
  note: DQ equations
  note: o1 equation
  reset : Inport
  u_d : Inport  Port=2
  u_q : Inport  Port=3
  u_o1 : Inport  Port=4
  u_o2 : Inport  Port=5
  u_x1 : Inport  Port=6
  u_y1 : Inport  Port=7
  u_x2 : Inport  Port=8
  u_y2 : Inport  Port=9
  u_zero : Inport  Port=10
  omega_mech : Inport  Port=11
  physical_parameters : Inport  Port=12
  Add{,1..6} (7 alike) : Sum  Inputs=+-
  Bus Selector : BusSelector  OutputSignals=1_L_d,1_L_q,R_1,polepair,psi_pm,L_z1,L_z2,L_x1,L_y1,L_x2,L_y2,L_z3
  Data Type Conversion{1..20,23} (21 alike) : DataTypeConversion  OutDataTypeStr=single  RndMeth=Nearest
  Data Type Conversion{21..22,24..30} (9 alike) : DataTypeConversion  OutDataTypeStr=double  RndMeth=Nearest
  Divide{,1..13} (14 alike) : Product  Inputs=**
  Product{,1,5..8,10} (7 alike) : Product
  Sum : Sum  Inputs=-++
  Sum1 : Sum  Inputs=-+-
  Sum2 : Sum  Inputs=-+|
  integrator : Subsystem
  integrator1 : Subsystem
  integrator2 : Subsystem
  integrator3 : Subsystem
  integrator4 : Subsystem
  integrator5 : Subsystem
  integrator6 : Subsystem
  integrator7 : Subsystem
  integrator8 : Subsystem
  I_d : Outport
  I_q : Outport  Port=2
  psi_d : Outport  Port=3
  psi_q : Outport  Port=4
  i_o1 : Outport  Port=5
  i_o2 : Outport  Port=6
  i_x1 : Outport  Port=7
  i_y1 : Outport  Port=8
  i_x2 : Outport  Port=9
  i_y2 : Outport  Port=10
  i_zero : Outport  Port=11
  tag scope: Reset=global
  wires:
  Data Type Conversion30/1 -> integrator8/1(in)
  Data Type Conversion29/1 -> integrator7/1(in)
  Data Type Conversion28/1 -> integrator6/1(in)
  Data Type Conversion27/1 -> integrator5/1(in)
  Data Type Conversion26/1 -> integrator4/1(in)
  Data Type Conversion25/1 -> integrator3/1(in)
  Data Type Conversion24/1 -> integrator2/1(in)
  Data Type Conversion22/1 -> integrator1/1(in)
  Data Type Conversion21/1 -> integrator/1(in)
  Data Type Conversion20/1 -> Divide13/1
  Data Type Conversion19/1 -> Divide11/1
  Data Type Conversion18/1 -> Divide9/1
  Data Type Conversion17/1 -> Divide7/1
  Data Type Conversion16/1 -> Divide5/1
  Data Type Conversion15/1 -> Divide3/1
  Data Type Conversion14/1 -> Divide1/1
  Data Type Conversion13/1 -> psi_q/1, Product/2, Product6/1
  Data Type Conversion23/1 -> Sum2/2, psi_d/1, Product1/2
  [L_z3] -> Divide13/2
  [L_y2] -> Divide11/2
  [L_x2] -> Divide9/2
  [L_y1] -> Divide7/2
  [L_x1] -> Divide5/2
  [polepairs] -> Product10/2
  Data Type Conversion2/1 -> [R1]
  Bus Selector/9 -> Data Type Conversion9/1  "<L_y1>"
  Data Type Conversion11/1 -> [reciprocal_Ld]
  Data Type Conversion3/1 -> [polepairs]
  physical_parameters/1 -> Bus Selector/1
  Data Type Conversion4/1 -> [L_z1]
  Bus Selector/10 -> Data Type Conversion8/1  "<L_x2>"
  Bus Selector/3 -> Data Type Conversion2/1  "<R_1>"
  Bus Selector/12 -> Data Type Conversion12/1  "<L_z3>"
  Bus Selector/11 -> Data Type Conversion10/1  "<L_y2>"
  Data Type Conversion6/1 -> [L_z2]
  Data Type Conversion7/1 -> [L_x1]
  Bus Selector/7 -> Data Type Conversion6/1  "<L_z2>"
  Bus Selector/6 -> Data Type Conversion4/1  "<L_z1>"
  Data Type Conversion10/1 -> [L_y2]
  Data Type Conversion8/1 -> [L_x2]
  Bus Selector/5 -> Data Type Conversion5/1  "<psi_pm>"
  Bus Selector/2 -> Data Type Conversion1/1  "<1_L_q>"
  Bus Selector/8 -> Data Type Conversion7/1  "<L_x1>"
  Bus Selector/4 -> Data Type Conversion3/1  "<polepair>"
  Data Type Conversion5/1 -> [psi_PM]
  Data Type Conversion1/1 -> [reciprocal_Lq]
  Data Type Conversion9/1 -> [L_y1]
  Data Type Conversion12/1 -> [L_z3]
  Bus Selector/1 -> Data Type Conversion11/1  "<1_L_d>"
  integrator8/1(outt) -> Data Type Conversion20/1  "psi_"
  [R1] -> Divide12/1
  Add6/1 -> Data Type Conversion30/1
  Divide12/1 -> Add6/2
  Divide13/1 -> Divide12/2, i_zero/1
  u_zero/1 -> Add6/1
  [Reset] -> integrator8/2(reset)
  [Reset] -> integrator7/2(reset)
  u_y2/1 -> Add5/1
  Divide11/1 -> Divide10/2, i_y2/1
  Divide10/1 -> Add5/2
  Add5/1 -> Data Type Conversion29/1
  [R1] -> Divide10/1
  integrator7/1(outt) -> Data Type Conversion19/1  "psi_"
  integrator6/1(outt) -> Data Type Conversion18/1  "psi_"
  [R1] -> Divide8/1
  Add4/1 -> Data Type Conversion28/1
  Divide8/1 -> Add4/2
  Divide9/1 -> Divide8/2, i_x2/1
  u_x2/1 -> Add4/1
  [Reset] -> integrator6/2(reset)
  [Reset] -> integrator5/2(reset)
  u_y1/1 -> Add3/1
  Divide7/1 -> Divide6/2, i_y1/1
  Divide6/1 -> Add3/2
  Add3/1 -> Data Type Conversion27/1
  [R1] -> Divide6/1
  integrator5/1(outt) -> Data Type Conversion17/1  "psi_"
  integrator4/1(outt) -> Data Type Conversion16/1  "psi_"
  [R1] -> Divide4/1
  Add2/1 -> Data Type Conversion26/1
  Divide4/1 -> Add2/2
  Divide5/1 -> Divide4/2, i_x1/1
  u_x1/1 -> Add2/1
  [Reset] -> integrator4/2(reset)
  [Reset] -> integrator3/2(reset)
  [L_z2] -> Divide3/2
  u_o2/1 -> Add1/1
  Divide3/1 -> Divide2/2, i_o2/1
  Divide2/1 -> Add1/2
  Add1/1 -> Data Type Conversion25/1
  [R1] -> Divide2/1
  integrator3/1(outt) -> Data Type Conversion15/1  "psi_"
  integrator2/1(outt) -> Data Type Conversion14/1  "psi_"
  [R1] -> Divide/1
  Add/1 -> Data Type Conversion24/1
  Divide/1 -> Add/2
  Divide1/1 -> Divide/2, i_o1/1
  u_o1/1 -> Add/1
  [L_z1] -> Divide1/2
  [Reset] -> integrator2/2(reset)
  [Reset] -> integrator1/2(reset)
  [Reset] -> integrator/2(reset)
  reset/1 -> [Reset]
  [R1] -> Product7/2
  [R1] -> Product8/2
  Sum1/1 -> Data Type Conversion22/1
  Product7/1 -> Sum1/3
  [reciprocal_Lq] -> Product6/2
  Product8/1 -> Sum/1
  Sum2/1 -> Product5/2
  integrator/1(outt) -> Data Type Conversion23/1  "psi_d"
  Product10/1 -> Product/1, Product1/1  "omega_el"
  Product6/1 -> Product7/1, I_q/1  "I_q"
  [psi_PM] -> Sum2/1
  Sum/1 -> Data Type Conversion21/1
  Product1/1 -> Sum1/1
  u_d/1 -> Sum/2
  integrator1/1(outt) -> Data Type Conversion13/1  "psi_q"
  [reciprocal_Ld] -> Product5/1
  Product5/1 -> Product8/1, I_d/1  "I_d"
  Product/1 -> Sum/3
  u_q/1 -> Sum1/2
  omega_mech/1 -> Product10/1

== system gm_uz_pmsm_model_9ph_working_vnl/uz_pmsm_model_9ph_vnl/torque_calculation ==
  I_d : Inport
  I_q : Inport  Port=2
  psi_d : Inport  Port=3
  psi_q : Inport  Port=4
  polepairs : Inport  Port=5
  Factor : Gain  Gain=9/2
  Product2 : Product
  Product3 : Product
  Product9 : Product
  Sum3 : Sum  Inputs=-|+
  M_Mi : Outport
  wires:
  Factor/1 -> Product9/1  "M_Mi"
  polepairs/1 -> Product9/2
  Product9/1 -> M_Mi/1  "M_Mi"
  I_q/1 -> Product3/2
  I_d/1 -> Product2/1
  psi_d/1 -> Product3/1
  psi_q/1 -> Product2/2
  Product2/1 -> Sum3/1
  Product3/1 -> Sum3/2
  Sum3/1 -> Factor/1

== system gm_uz_pmsm_model_9ph_working_vnl/Compare/Assert_i_dq_ps/RelErrCheck ==
  In1 : Inport
  In2 : Inport  Port=2
  "RelativeErrorCheck " : MATLAB Function  TreatAsAtomicUnit=on
  Out1 : Outport  VectorParamsAs1DForOutWhenUnconnected=off
  wires:
  "RelativeErrorCheck "/1(y) -> Out1/1
  In1/1 -> "RelativeErrorCheck "/1(P)
  In2/1 -> "RelativeErrorCheck "/2(R)

== system gm_uz_pmsm_model_9ph_working_vnl/Compare/Assert_outputs/RelErrCheck ==
  In1 : Inport
  In2 : Inport  Port=2
  "RelativeErrorCheck " : MATLAB Function  TreatAsAtomicUnit=on
  Out1 : Outport  VectorParamsAs1DForOutWhenUnconnected=off
  wires:
  "RelativeErrorCheck "/1(y) -> Out1/1
  In1/1 -> "RelativeErrorCheck "/1(P)
  In2/1 -> "RelativeErrorCheck "/2(R)

== system gm_uz_pmsm_model_9ph_working_vnl/uz_pmsm_model_9ph/Theta_el/Data Type Conversion1 ==
  In1 : Inport
  Data Type Conversion1 : DataTypeConversion  OutDataTypeStr=single  RndMeth=Nearest  SampleTime=2e-09
  Data Type Conversion1_pd1 : Delay  DelayLength=3
  Out1 : Outport
  wires:
  Data Type Conversion1_pd1/1 -> Out1/1
  Data Type Conversion1/1 -> Data Type Conversion1_pd1/1
  In1/1 -> Data Type Conversion1/1

== system gm_uz_pmsm_model_9ph_working_vnl/uz_pmsm_model_9ph/Theta_el/Data Type Conversion2 ==
  In1 : Inport
  Data Type Conversion2 : DataTypeConversion  OutDataTypeStr=double  RndMeth=Nearest  SampleTime=2e-09
  Data Type Conversion2_pd1 : Delay  DelayLength=3
  Out1 : Outport
  wires:
  Data Type Conversion2_pd1/1 -> Out1/1
  Data Type Conversion2/1 -> Data Type Conversion2_pd1/1
  In1/1 -> Data Type Conversion2/1

== system gm_uz_pmsm_model_9ph_working_vnl/uz_pmsm_model_9ph/Theta_el/Divide ==
  In1 : Inport
  In2 : Inport  Port=2
  Divide : Product  Inputs=**  OutDataTypeStr=single  SampleTime=2e-09
  Divide_pd1 : Delay  DelayLength=6
  Out1 : Outport
  wires:
  Divide_pd1/1 -> Out1/1
  Divide/1 -> Divide_pd1/1
  In2/1 -> Divide/2
  In1/1 -> Divide/1

== system gm_uz_pmsm_model_9ph_working_vnl/uz_pmsm_model_9ph/Theta_el/Gain ==
  In1 : Inport
  In2 : Inport  Port=2
  Gain : Product  Inputs=**  OutDataTypeStr=double  SampleTime=2e-09
  Gain_pd1 : Delay  DelayLength=6
  Out1 : Outport
  wires:
  Gain_pd1/1 -> Out1/1
  Gain/1 -> Gain_pd1/1
  In2/1 -> Gain/2
  In1/1 -> Gain/1

== system gm_uz_pmsm_model_9ph_working_vnl/uz_pmsm_model_9ph/Theta_el/Mod ==
  In1 : Inport
  In2 : Inport  Port=2
  Mod : Math  Operator=rem  SampleTime=2e-09  SaturateOnIntegerOverflow=on
  Mod_pd1 : Delay  DelayLength=15
  Out1 : Outport
  wires:
  Mod_pd1/1 -> Out1/1
  Mod/1 -> Mod_pd1/1
  In2/1 -> Mod/2
  In1/1 -> Mod/1

== system gm_uz_pmsm_model_9ph_working_vnl/uz_pmsm_model_9ph/Theta_el/Sum3 ==
  In1 : Inport
  In2 : Inport  Port=2
  Sum3 : Sum  OutDataTypeStr=double  SampleTime=2e-09
  Sum3_pd1 : Delay  DelayLength=6
  Out1 : Outport
  wires:
  Sum3_pd1/1 -> Out1/1
  Sum3/1 -> Sum3_pd1/1
  In2/1 -> Sum3/2
  In1/1 -> Sum3/1

== system gm_uz_pmsm_model_9ph_working_vnl/uz_pmsm_model_9ph/Transformation/Add ==
  In1 : Inport
  In2 : Inport  Port=2
  Add : Sum  OutDataTypeStr=single  SampleTime=2e-09
  Add_pd1 : Delay  DelayLength=6
  Out1 : Outport
  wires:
  Add_pd1/1 -> Out1/1
  Add/1 -> Add_pd1/1
  In2/1 -> Add/2
  In1/1 -> Add/1

== system gm_uz_pmsm_model_9ph_working_vnl/uz_pmsm_model_9ph/Transformation/Add1 ==
  In1 : Inport
  In2 : Inport  Port=2
  Add1 : Sum  Inputs=+-  OutDataTypeStr=single  SampleTime=2e-09
  Add1_pd1 : Delay  DelayLength=6
  Out1 : Outport
  wires:
  Add1_pd1/1 -> Out1/1
  Add1/1 -> Add1_pd1/1
  In2/1 -> Add1/2
  In1/1 -> Add1/1

== system gm_uz_pmsm_model_9ph_working_vnl/uz_pmsm_model_9ph/Transformation/Data Type Conversion39 ==
  In1 : Inport
  Data Type Conversion39 : DataTypeConversion  OutDataTypeStr=single  RndMeth=Nearest  SampleTime=2e-09
  Data Type Conversion39_pd1 : Delay  DelayLength=6
  Out1 : Outport
  wires:
  Data Type Conversion39_pd1/1 -> Out1/1
  Data Type Conversion39/1 -> Data Type Conversion39_pd1/1
  In1/1 -> Data Type Conversion39/1

== system gm_uz_pmsm_model_9ph_working_vnl/uz_pmsm_model_9ph/Transformation/Divide ==
  In1 : Inport
  In2 : Inport  Port=2
  Divide : Product  Inputs=**  OutDataTypeStr=single  SampleTime=2e-09
  Divide_pd1 : Delay  DelayLength=6
  Out1 : Outport
  wires:
  Divide_pd1/1 -> Out1/1
  Divide/1 -> Divide_pd1/1
  In2/1 -> Divide/2
  In1/1 -> Divide/1

== system gm_uz_pmsm_model_9ph_working_vnl/uz_pmsm_model_9ph/Transformation/Divide1 ==
  In1 : Inport
  In2 : Inport  Port=2
  Divide1 : Product  Inputs=**  OutDataTypeStr=single  SampleTime=2e-09
  Divide1_pd1 : Delay  DelayLength=6
  Out1 : Outport
  wires:
  Divide1_pd1/1 -> Out1/1
  Divide1/1 -> Divide1_pd1/1
  In2/1 -> Divide1/2
  In1/1 -> Divide1/1

== system gm_uz_pmsm_model_9ph_working_vnl/uz_pmsm_model_9ph/Transformation/Divide2 ==
  In1 : Inport
  In2 : Inport  Port=2
  Divide2 : Product  Inputs=**  OutDataTypeStr=single  SampleTime=2e-09
  Divide2_pd1 : Delay  DelayLength=6
  Out1 : Outport
  wires:
  Divide2_pd1/1 -> Out1/1
  Divide2/1 -> Divide2_pd1/1
  In2/1 -> Divide2/2
  In1/1 -> Divide2/1

== system gm_uz_pmsm_model_9ph_working_vnl/uz_pmsm_model_9ph/Transformation/Divide3 ==
  In1 : Inport
  In2 : Inport  Port=2
  Divide3 : Product  Inputs=**  OutDataTypeStr=single  SampleTime=2e-09
  Divide3_pd1 : Delay  DelayLength=6
  Out1 : Outport
  wires:
  Divide3_pd1/1 -> Out1/1
  Divide3/1 -> Divide3_pd1/1
  In2/1 -> Divide3/2
  In1/1 -> Divide3/1

== system gm_uz_pmsm_model_9ph_working_vnl/uz_pmsm_model_9ph/Transformation/t3 ==
  in0 : Inport
  ColVec1 : Selector  NumberOfDimensions=2  IndexOptions=Select all,Index vector (dialog)  Indices=1,1  OutputSizes=1,1
  ColVec2 : Selector  NumberOfDimensions=2  IndexOptions=Select all,Index vector (dialog)  Indices=1,2  OutputSizes=1,1
  ColVec3 : Selector  NumberOfDimensions=2  IndexOptions=Select all,Index vector (dialog)  Indices=1,3  OutputSizes=1,1
  ColVec4 : Selector  NumberOfDimensions=2  IndexOptions=Select all,Index vector (dialog)  Indices=1,4  OutputSizes=1,1
  ColVec5 : Selector  NumberOfDimensions=2  IndexOptions=Select all,Index vector (dialog)  Indices=1,5  OutputSizes=1,1
  ColVec6 : Selector  NumberOfDimensions=2  IndexOptions=Select all,Index vector (dialog)  Indices=1,6  OutputSizes=1,1
  ColVec7 : Selector  NumberOfDimensions=2  IndexOptions=Select all,Index vector (dialog)  Indices=1,7  OutputSizes=1,1
  ColVec8 : Selector  NumberOfDimensions=2  IndexOptions=Select all,Index vector (dialog)  Indices=1,8  OutputSizes=1,1
  ColVec9 : Selector  NumberOfDimensions=2  IndexOptions=Select all,Index vector (dialog)  Indices=1,9  OutputSizes=1,1
  out0 : Outport
  out1 : Outport  Port=2
  out2 : Outport  Port=3
  out3 : Outport  Port=4
  out4 : Outport  Port=5
  out5 : Outport  Port=6
  out6 : Outport  Port=7
  out7 : Outport  Port=8
  out8 : Outport  Port=9
  wires:
  ColVec9/1 -> out8/1
  ColVec8/1 -> out7/1
  ColVec7/1 -> out6/1
  ColVec6/1 -> out5/1
  ColVec5/1 -> out4/1
  ColVec4/1 -> out3/1
  ColVec3/1 -> out2/1
  ColVec2/1 -> out1/1
  ColVec1/1 -> out0/1
  in0/1 -> ColVec9/1, ColVec8/1, ColVec7/1, ColVec6/1, ColVec5/1, ColVec4/1, ColVec3/1, ColVec2/1, ColVec1/1

== system gm_uz_pmsm_model_9ph_working_vnl/uz_pmsm_model_9ph/Transformation1/Add ==
  In1 : Inport
  In2 : Inport  Port=2
  Add : Sum  Inputs=+-  OutDataTypeStr=single  SampleTime=2e-09
  Add_pd1 : Delay  DelayLength=6
  Out1 : Outport
  wires:
  Add_pd1/1 -> Out1/1
  Add/1 -> Add_pd1/1
  In2/1 -> Add/2
  In1/1 -> Add/1

== system gm_uz_pmsm_model_9ph_working_vnl/uz_pmsm_model_9ph/Transformation1/Add1 ==
  In1 : Inport
  In2 : Inport  Port=2
  Add1 : Sum  OutDataTypeStr=single  SampleTime=2e-09
  Add1_pd1 : Delay  DelayLength=6
  Out1 : Outport
  wires:
  Add1_pd1/1 -> Out1/1
  Add1/1 -> Add1_pd1/1
  In2/1 -> Add1/2
  In1/1 -> Add1/1

== system gm_uz_pmsm_model_9ph_working_vnl/uz_pmsm_model_9ph/Transformation1/Data Type Conversion28 ==
  In1 : Inport
  Data Type Conversion28 : DataTypeConversion  OutDataTypeStr=fixdt(1, 25, 12)  RndMeth=Nearest  SampleTime=2e-09
  Data Type Conversion28_pd1 : Delay  DelayLength=6
  Out1 : Outport
  wires:
  Data Type Conversion28_pd1/1 -> Out1/1
  Data Type Conversion28/1 -> Data Type Conversion28_pd1/1
  In1/1 -> Data Type Conversion28/1

== system gm_uz_pmsm_model_9ph_working_vnl/uz_pmsm_model_9ph/Transformation1/Divide ==
  In1 : Inport
  In2 : Inport  Port=2
  Divide : Product  Inputs=**  OutDataTypeStr=single  SampleTime=2e-09
  Divide_pd1 : Delay  DelayLength=6
  Out1 : Outport
  wires:
  Divide_pd1/1 -> Out1/1
  Divide/1 -> Divide_pd1/1
  In2/1 -> Divide/2
  In1/1 -> Divide/1

== system gm_uz_pmsm_model_9ph_working_vnl/uz_pmsm_model_9ph/Transformation1/Divide1 ==
  In1 : Inport
  In2 : Inport  Port=2
  Divide1 : Product  Inputs=**  OutDataTypeStr=single  SampleTime=2e-09
  Divide1_pd1 : Delay  DelayLength=6
  Out1 : Outport
  wires:
  Divide1_pd1/1 -> Out1/1
  Divide1/1 -> Divide1_pd1/1
  In2/1 -> Divide1/2
  In1/1 -> Divide1/1

== system gm_uz_pmsm_model_9ph_working_vnl/uz_pmsm_model_9ph/Transformation1/Divide2 ==
  In1 : Inport
  In2 : Inport  Port=2
  Divide2 : Product  Inputs=**  OutDataTypeStr=single  SampleTime=2e-09
  Divide2_pd1 : Delay  DelayLength=6
  Out1 : Outport
  wires:
  Divide2_pd1/1 -> Out1/1
  Divide2/1 -> Divide2_pd1/1
  In2/1 -> Divide2/2
  In1/1 -> Divide2/1

== system gm_uz_pmsm_model_9ph_working_vnl/uz_pmsm_model_9ph/Transformation1/Divide3 ==
  In1 : Inport
  In2 : Inport  Port=2
  Divide3 : Product  Inputs=**  OutDataTypeStr=single  SampleTime=2e-09
  Divide3_pd1 : Delay  DelayLength=6
  Out1 : Outport
  wires:
  Divide3_pd1/1 -> Out1/1
  Divide3/1 -> Divide3_pd1/1
  In2/1 -> Divide3/2
  In1/1 -> Divide3/1

== system gm_uz_pmsm_model_9ph_working_vnl/uz_pmsm_model_9ph/Transformation1/Transformation1_MAC ==
  in0 : Inport  OutDataTypeStr=fixdt(1, 18, 16)  PortDimensions=[9 1]  SampleTime=2e-09
  in1 : Inport  Port=2  OutDataTypeStr=fixdt(1, 25, 12)  PortDimensions=[9]  SampleTime=2e-09
  globalSchedule : EnablePort  OutDataTypeStr=boolean
  PipelineRegister : Delay  DelayLength=double(8)  InitialCondition=0
  t : hdlsllib/HDL Operations/Multiply-Accumulate  opMode=Vector  initValueSetting=Dialog  initValue=0  initValueSetting2=Dialog  initValue2=0  initValueSetting3=Dialog  initValue3=0  num_samples=2  RndMeth2=Floor  RndMeth3=Floor  OutDataTypeStr=fixdt(1, 43, 28)  datatype2=Inherit: Inherit via back propagation  datatype3=Inherit: Inherit via back propagation  validOut=on  endInandOut=on  startOut=on  countOut=on  dim=-1  DoSatur=off  parallel=off
      settings: SourceProductBaseCode=SL
  out0 : Outport  OutDataTypeStr=fixdt(1, 43, 28)  SampleTime=2e-09  InitialOutput=0
  wires:
  t/1 -> PipelineRegister/1
  in1/1 -> t/2
  in0/1 -> t/1
  PipelineRegister/1 -> out0/1

== system gm_uz_pmsm_model_9ph_working_vnl/uz_pmsm_model_9ph/Transformation1/Transformation1_MAC1 ==
  in0 : Inport  OutDataTypeStr=fixdt(1, 18, 16)  PortDimensions=[9 1]  SampleTime=2e-09
  in1 : Inport  Port=2  OutDataTypeStr=fixdt(1, 25, 12)  PortDimensions=[9]  SampleTime=2e-09
  globalSchedule : EnablePort  OutDataTypeStr=boolean
  PipelineRegister : Delay  DelayLength=double(8)  InitialCondition=0
  t : hdlsllib/HDL Operations/Multiply-Accumulate  opMode=Vector  initValueSetting=Dialog  initValue=0  initValueSetting2=Dialog  initValue2=0  initValueSetting3=Dialog  initValue3=0  num_samples=2  RndMeth2=Floor  RndMeth3=Floor  OutDataTypeStr=fixdt(1, 43, 28)  datatype2=Inherit: Inherit via back propagation  datatype3=Inherit: Inherit via back propagation  validOut=on  endInandOut=on  startOut=on  countOut=on  dim=-1  DoSatur=off  parallel=off
      settings: SourceProductBaseCode=SL
  out0 : Outport  OutDataTypeStr=fixdt(1, 43, 28)  SampleTime=2e-09  InitialOutput=0
  wires:
  t/1 -> PipelineRegister/1
  in1/1 -> t/2
  in0/1 -> t/1
  PipelineRegister/1 -> out0/1

== system gm_uz_pmsm_model_9ph_working_vnl/uz_pmsm_model_9ph/Transformation1/Transformation1_MAC2 ==
  in0 : Inport  OutDataTypeStr=fixdt(1, 18, 16)  PortDimensions=[9 1]  SampleTime=2e-09
  in1 : Inport  Port=2  OutDataTypeStr=fixdt(1, 25, 12)  PortDimensions=[9]  SampleTime=2e-09
  globalSchedule : EnablePort  OutDataTypeStr=boolean
  PipelineRegister : Delay  DelayLength=double(8)  InitialCondition=0
  t : hdlsllib/HDL Operations/Multiply-Accumulate  opMode=Vector  initValueSetting=Dialog  initValue=0  initValueSetting2=Dialog  initValue2=0  initValueSetting3=Dialog  initValue3=0  num_samples=2  RndMeth2=Floor  RndMeth3=Floor  OutDataTypeStr=fixdt(1, 43, 28)  datatype2=Inherit: Inherit via back propagation  datatype3=Inherit: Inherit via back propagation  validOut=on  endInandOut=on  startOut=on  countOut=on  dim=-1  DoSatur=off  parallel=off
      settings: SourceProductBaseCode=SL
  out0 : Outport  OutDataTypeStr=fixdt(1, 43, 28)  SampleTime=2e-09  InitialOutput=0
  wires:
  t/1 -> PipelineRegister/1
  in1/1 -> t/2
  in0/1 -> t/1
  PipelineRegister/1 -> out0/1

== system gm_uz_pmsm_model_9ph_working_vnl/uz_pmsm_model_9ph/Transformation1/Transformation1_MAC3 ==
  in0 : Inport  OutDataTypeStr=fixdt(1, 18, 16)  PortDimensions=[9 1]  SampleTime=2e-09
  in1 : Inport  Port=2  OutDataTypeStr=fixdt(1, 25, 12)  PortDimensions=[9]  SampleTime=2e-09
  globalSchedule : EnablePort  OutDataTypeStr=boolean
  PipelineRegister : Delay  DelayLength=double(8)  InitialCondition=0
  t : hdlsllib/HDL Operations/Multiply-Accumulate  opMode=Vector  initValueSetting=Dialog  initValue=0  initValueSetting2=Dialog  initValue2=0  initValueSetting3=Dialog  initValue3=0  num_samples=2  RndMeth2=Floor  RndMeth3=Floor  OutDataTypeStr=fixdt(1, 43, 28)  datatype2=Inherit: Inherit via back propagation  datatype3=Inherit: Inherit via back propagation  validOut=on  endInandOut=on  startOut=on  countOut=on  dim=-1  DoSatur=off  parallel=off
      settings: SourceProductBaseCode=SL
  out0 : Outport  OutDataTypeStr=fixdt(1, 43, 28)  SampleTime=2e-09  InitialOutput=0
  wires:
  t/1 -> PipelineRegister/1
  in1/1 -> t/2
  in0/1 -> t/1
  PipelineRegister/1 -> out0/1

== system gm_uz_pmsm_model_9ph_working_vnl/uz_pmsm_model_9ph/Transformation1/Transformation1_MAC4 ==
  in0 : Inport  OutDataTypeStr=fixdt(1, 18, 16)  PortDimensions=[9 1]  SampleTime=2e-09
  in1 : Inport  Port=2  OutDataTypeStr=fixdt(1, 25, 12)  PortDimensions=[9]  SampleTime=2e-09
  globalSchedule : EnablePort  OutDataTypeStr=boolean
  PipelineRegister : Delay  DelayLength=double(8)  InitialCondition=0
  t : hdlsllib/HDL Operations/Multiply-Accumulate  opMode=Vector  initValueSetting=Dialog  initValue=0  initValueSetting2=Dialog  initValue2=0  initValueSetting3=Dialog  initValue3=0  num_samples=2  RndMeth2=Floor  RndMeth3=Floor  OutDataTypeStr=fixdt(1, 43, 28)  datatype2=Inherit: Inherit via back propagation  datatype3=Inherit: Inherit via back propagation  validOut=on  endInandOut=on  startOut=on  countOut=on  dim=-1  DoSatur=off  parallel=off
      settings: SourceProductBaseCode=SL
  out0 : Outport  OutDataTypeStr=fixdt(1, 43, 28)  SampleTime=2e-09  InitialOutput=0
  wires:
  t/1 -> PipelineRegister/1
  in1/1 -> t/2
  in0/1 -> t/1
  PipelineRegister/1 -> out0/1

== system gm_uz_pmsm_model_9ph_working_vnl/uz_pmsm_model_9ph/Transformation1/Transformation1_MAC5 ==
  in0 : Inport  OutDataTypeStr=fixdt(1, 18, 16)  PortDimensions=[9 1]  SampleTime=2e-09
  in1 : Inport  Port=2  OutDataTypeStr=fixdt(1, 25, 12)  PortDimensions=[9]  SampleTime=2e-09
  globalSchedule : EnablePort  OutDataTypeStr=boolean
  PipelineRegister : Delay  DelayLength=double(8)  InitialCondition=0
  t : hdlsllib/HDL Operations/Multiply-Accumulate  opMode=Vector  initValueSetting=Dialog  initValue=0  initValueSetting2=Dialog  initValue2=0  initValueSetting3=Dialog  initValue3=0  num_samples=2  RndMeth2=Floor  RndMeth3=Floor  OutDataTypeStr=fixdt(1, 43, 28)  datatype2=Inherit: Inherit via back propagation  datatype3=Inherit: Inherit via back propagation  validOut=on  endInandOut=on  startOut=on  countOut=on  dim=-1  DoSatur=off  parallel=off
      settings: SourceProductBaseCode=SL
  out0 : Outport  OutDataTypeStr=fixdt(1, 43, 28)  SampleTime=2e-09  InitialOutput=0
  wires:
  t/1 -> PipelineRegister/1
  in1/1 -> t/2
  in0/1 -> t/1
  PipelineRegister/1 -> out0/1

== system gm_uz_pmsm_model_9ph_working_vnl/uz_pmsm_model_9ph/Transformation1/Transformation1_MAC6 ==
  in0 : Inport  OutDataTypeStr=fixdt(1, 18, 16)  PortDimensions=[9 1]  SampleTime=2e-09
  in1 : Inport  Port=2  OutDataTypeStr=fixdt(1, 25, 12)  PortDimensions=[9]  SampleTime=2e-09
  globalSchedule : EnablePort  OutDataTypeStr=boolean
  PipelineRegister : Delay  DelayLength=double(8)  InitialCondition=0
  t : hdlsllib/HDL Operations/Multiply-Accumulate  opMode=Vector  initValueSetting=Dialog  initValue=0  initValueSetting2=Dialog  initValue2=0  initValueSetting3=Dialog  initValue3=0  num_samples=2  RndMeth2=Floor  RndMeth3=Floor  OutDataTypeStr=fixdt(1, 43, 28)  datatype2=Inherit: Inherit via back propagation  datatype3=Inherit: Inherit via back propagation  validOut=on  endInandOut=on  startOut=on  countOut=on  dim=-1  DoSatur=off  parallel=off
      settings: SourceProductBaseCode=SL
  out0 : Outport  OutDataTypeStr=fixdt(1, 43, 28)  SampleTime=2e-09  InitialOutput=0
  wires:
  t/1 -> PipelineRegister/1
  in1/1 -> t/2
  in0/1 -> t/1
  PipelineRegister/1 -> out0/1

== system gm_uz_pmsm_model_9ph_working_vnl/uz_pmsm_model_9ph/Transformation1/Transformation1_MAC7 ==
  in0 : Inport  OutDataTypeStr=fixdt(1, 18, 16)  PortDimensions=[9 1]  SampleTime=2e-09
  in1 : Inport  Port=2  OutDataTypeStr=fixdt(1, 25, 12)  PortDimensions=[9]  SampleTime=2e-09
  globalSchedule : EnablePort  OutDataTypeStr=boolean
  PipelineRegister : Delay  DelayLength=double(8)  InitialCondition=0
  t : hdlsllib/HDL Operations/Multiply-Accumulate  opMode=Vector  initValueSetting=Dialog  initValue=0  initValueSetting2=Dialog  initValue2=0  initValueSetting3=Dialog  initValue3=0  num_samples=2  RndMeth2=Floor  RndMeth3=Floor  OutDataTypeStr=fixdt(1, 43, 28)  datatype2=Inherit: Inherit via back propagation  datatype3=Inherit: Inherit via back propagation  validOut=on  endInandOut=on  startOut=on  countOut=on  dim=-1  DoSatur=off  parallel=off
      settings: SourceProductBaseCode=SL
  out0 : Outport  OutDataTypeStr=fixdt(1, 43, 28)  SampleTime=2e-09  InitialOutput=0
  wires:
  t/1 -> PipelineRegister/1
  in1/1 -> t/2
  in0/1 -> t/1
  PipelineRegister/1 -> out0/1
